simulink model "CRDI_Integrated_Model0707"  (R2019a)
settings: configuration reference "cs1" (kept outside this file)
PreLoadFcn:
  | Configaration_Setting
settings Model: DataDictionary=CRDI_Integrated_Model.sldd  EnableAccessToBaseWorkspace=off  Creator=ADVAIT ELECTRICALS  LastModifiedBy=ADVAIT ELECTRICALS
settings ConfigSetRef: SourceName=cs1

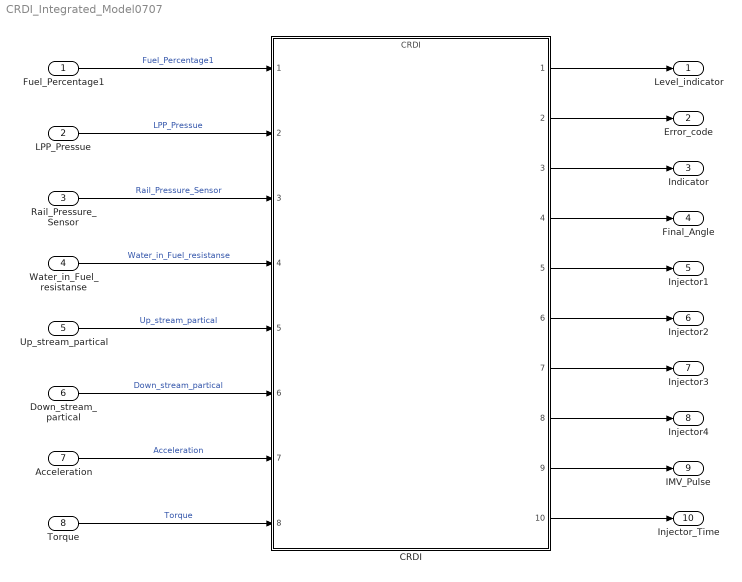
== system CRDI_Integrated_Model0707 ==
  Fuel_Percentage1 : Inport
  LPP_Pressue : Inport  Port=2
  Rail_Pressure_Sensor : Inport  Port=3
  Water_in_Fuel_resistanse : Inport  Port=4
  Up_stream_partical : Inport  Port=5
  Down_stream_partical : Inport  Port=6
  Acceleration : Inport  Port=7
  Torque : Inport  Port=8
  CRDI : ModelReference  ModelNameDialog=CRDI  SimulationMode=Normal  ModelReferenceVersion=1.42
  Level_indicator : Outport
  Error_code : Outport  Port=2
  Indicator : Outport  Port=3
  Final_Angle : Outport  Port=4
  Injector1 : Outport  Port=5
  Injector2 : Outport  Port=6
  Injector3 : Outport  Port=7
  Injector4 : Outport  Port=8
  IMV_Pulse : Outport  Port=9
  Injector_Time : Outport  Port=10
  wires:
  LPP_Pressue/1 -> CRDI/2  "LPP_Pressue"
  Fuel_Percentage1/1 -> CRDI/1  "Fuel_Percentage1"
  Rail_Pressure_Sensor/1 -> CRDI/3  "Rail_Pressure_Sensor"
  Up_stream_partical/1 -> CRDI/5  "Up_stream_partical"
  Water_in_Fuel_resistanse/1 -> CRDI/4  "Water_in_Fuel_resistanse"
  Down_stream_partical/1 -> CRDI/6  "Down_stream_partical"
  CRDI/1 -> Level_indicator/1
  CRDI/2 -> Error_code/1
  CRDI/3 -> Indicator/1
  CRDI/6 -> Injector2/1
  CRDI/5 -> Injector1/1
  CRDI/4 -> Final_Angle/1
  CRDI/9 -> IMV_Pulse/1
  CRDI/10 -> Injector_Time/1
  CRDI/8 -> Injector4/1
  CRDI/7 -> Injector3/1
  Acceleration/1 -> CRDI/7  "Acceleration"
  Torque/1 -> CRDI/8  "Torque"
